simulink model "Beschl_self_geschaltet"  (R2021a)
settings: Solver=VariableStepAuto  StartTime=0.0  StopTime=20  RelTol=1e-3
values from neighbouring files (symbols this model uses):
  A = 1.7    [Parameter_Beschleunigen_Rueckschaltung.m]
  c_W = 0.32    [Parameter_Beschleunigen_Rueckschaltung.m]
  eta = 0.9    [Parameter_Beschleunigen_Rueckschaltung.m]
  F_R = 160    [Parameter_Beschleunigen_Rueckschaltung.m]
  i_A = 4.06    [Parameter_Beschleunigen_Rueckschaltung.m]
  i_G5 = 1.3    [Parameter_Beschleunigen_Rueckschaltung.m]
  m = 1600    [Parameter_Beschleunigen_Rueckschaltung.m]
  r_R = 0.291    [Parameter_Beschleunigen_Rueckschaltung.m]
  rho = 1.2    [Parameter_Beschleunigen_Rueckschaltung.m]
  v_0 = 60/3.6    (= 16.6666666667)    [Parameter_Beschleunigen_Rueckschaltung.m]
  v_max = r_R * omega_Rad_max    (= 37.5288777584)    [Parameter_Beschleunigen_Rueckschaltung.m]
  v_max_4 = r_R * omega_Rad_max_4    (= 23.2321624219)    [Parameter_Beschleunigen_Rueckschaltung.m]
libraries: simulink x2
settings Model: Creator=Kempk  LastModifiedBy=Kempk

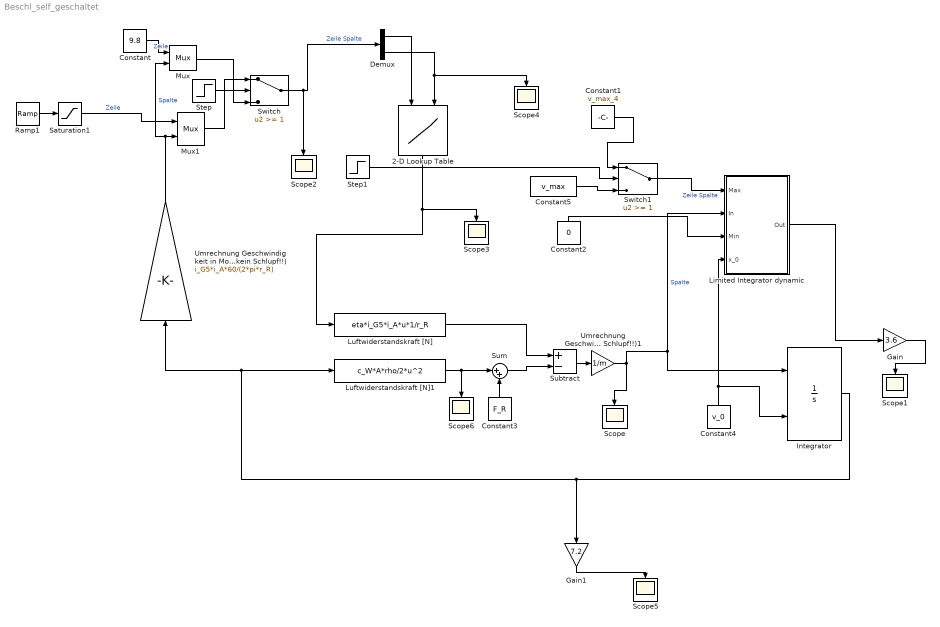
== system Beschl_self_geschaltet ==
  2-D Lookup Table : Lookup_n-D  BreakpointsForDimension1=KF_Motor(2:end,1)  BreakpointsForDimension2=KF_Motor(1,2:end)  Table=KF_Motor(2:end,2:end)  InternalRulePriority=Speed  RndMeth=Simplest  InputSameDT=on
      settings: InputPortMap=u0,u1
  Constant : Constant  Value=9.8
  Constant1 : Constant  Value=v_max_4
  Constant2 : Constant  Value=0
  Constant3 : Constant  Value=F_R
  Constant4 : Constant  Value=v_0
  Constant5 : Constant  Value=v_max
  Demux : Demux  Outputs=2
  Gain : Gain  Gain=3.6
  Gain1 : Gain  Gain=7.2
  Integrator : Integrator  InitialConditionSource=external  LimitOutput=on  UpperSaturationLimit=v_max
  Limited Integrator dynamic : Subsystem
  Luftwiderstandskraft [N] : Fcn  Expr=eta*i_G5*i_A*u*1/r_R
  Luftwiderstandskraft [N]1 : Fcn  Expr=c_W*A*rho/2*u^2
  Mux : Mux  Inputs=2
      settings: DisplayOption=signals
  Mux1 : Mux  Inputs=2
      settings: DisplayOption=signals
  Ramp1 : simulink/Sources/Ramp  slope=5000  start=3  InitialOutput=9.8
  Saturation1 : Saturate  UpperLimit=90  LowerLimit=9.8
  Scope{,1..6} (7 alike) : Scope
  Step : Step  Time=3  SampleTime=0
  Step1 : Step  Time=5  SampleTime=0
  Subtract : Sum  Inputs=+-
  Sum : Sum  Inputs=|++
  Switch : Switch  Threshold=1
  Switch1 : Switch  Threshold=1
  Umrechnung Geschwindigkeit in Motordrehzahl (kein Schlupf!!) : Gain  Gain=i_G5*i_A*60/(2*pi*r_R)
  Umrechnung Geschwindigkeit in Motordrehzahl (kein Schlupf!!)1 : Gain  Gain=1/m
  wires:
  Step/1 -> Switch/2
  Switch/1 -> Demux/1, Scope2/1  "Zeile Spalte"
  Luftwiderstandskraft [N]1/1 -> Sum/1, Scope6/1
  Constant3/1 -> Sum/2
  Sum/1 -> Subtract/2
  Luftwiderstandskraft [N]/1 -> Subtract/1
  2-D Lookup Table/1 -> Scope3/1, Luftwiderstandskraft [N]/1
  Integrator/1 -> Gain1/1, Umrechnung Geschwindigkeit in Motordrehzahl (kein Schlupf!!)/1, Luftwiderstandskraft [N]1/1
  Constant4/1 -> Limited Integrator dynamic/4(x_0), Integrator/2
  Constant/1 -> Mux/1  "Zeile"
  Saturation1/1 -> Mux1/1  "Zeile"
  Umrechnung Geschwindigkeit in Motordrehzahl (kein Schlupf!!)/1 -> Mux/2, Mux1/2  "Spalte"
  Demux/1 -> 2-D Lookup Table/1
  Demux/2 -> Scope4/1, 2-D Lookup Table/2
  Mux/1 -> Switch/3
  Mux1/1 -> Switch/1
  Gain/1 -> Scope1/1
  Ramp1/1 -> Saturation1/1
  Subtract/1 -> Umrechnung Geschwindigkeit in Motordrehzahl (kein Schlupf!!)1/1
  Umrechnung Geschwindigkeit in Motordrehzahl (kein Schlupf!!)1/1 -> Scope/1, Limited Integrator dynamic/2(In), Integrator/1  "Spalte"
  Limited Integrator dynamic/1(Out) -> Gain/1
  Constant2/1 -> Limited Integrator dynamic/3(Min)
  Step1/1 -> Switch1/2
  Switch1/1 -> Limited Integrator dynamic/1(Max)  "Zeile Spalte"
  Constant1/1 -> Switch1/1
  Constant5/1 -> Switch1/3
  Gain1/1 -> Scope5/1

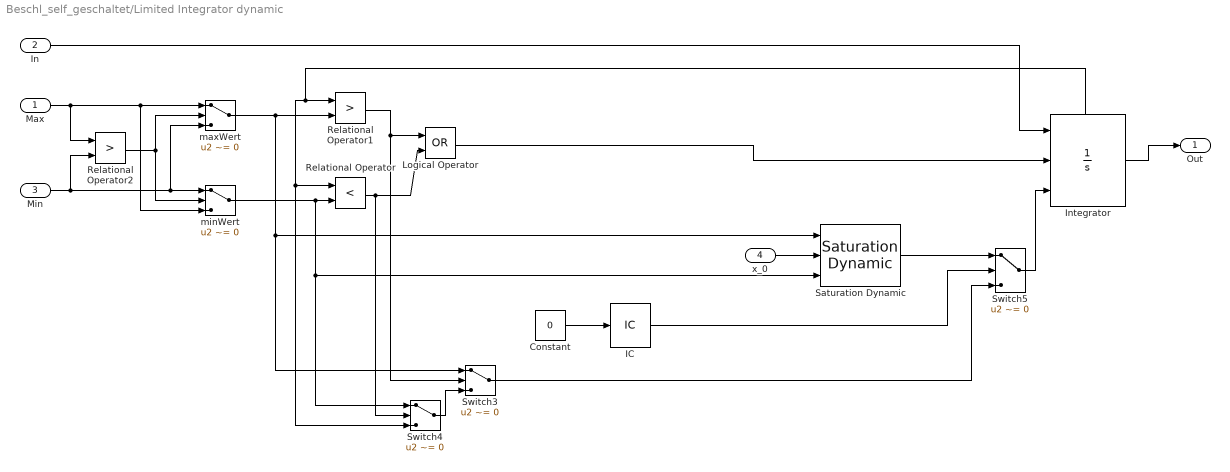
== system Beschl_self_geschaltet/Limited Integrator dynamic ==
  Max : Inport
  In : Inport  Port=2
  Min : Inport  Port=3
  x_0 : Inport  Port=4
  Constant : Constant  Value=0
  IC : InitialCondition
  Integrator : Integrator  ExternalReset=level  InitialConditionSource=external  ShowStatePort=on
  Logical Operator : Logic  Operator=OR  AllPortsSameDT=off  OutDataTypeStr=boolean
  Relational Operator : RelationalOperator  Operator=<  OutDataTypeStr=boolean  RndMeth=Nearest
  Relational Operator1 : RelationalOperator  Operator=>  OutDataTypeStr=boolean  RndMeth=Nearest
  Relational Operator2 : RelationalOperator  Operator=>  OutDataTypeStr=boolean  RndMeth=Nearest
  Saturation Dynamic : simulink/Discontinuities/Saturation Dynamic  OutMin=[]  OutMax=[]  OutDataTypeStr=Inherit: Same as second input  OutDataType=fixdt(1, 16)  OutScaling=2^-10  DoSatur=off
  Switch3 : Switch  Criteria=u2 ~= 0
  Switch4 : Switch  Criteria=u2 ~= 0
  Switch5 : Switch  Criteria=u2 ~= 0
  maxWert : Switch  Criteria=u2 ~= 0
  minWert : Switch  Criteria=u2 ~= 0
  Out : Outport
  wires:
  Integrator/1 -> Out/1
  maxWert/1 -> Relational Operator1/2, Switch3/1, Saturation Dynamic/1
  minWert/1 -> Relational Operator/2, Switch4/1, Saturation Dynamic/3
  Relational Operator1/1 -> Logical Operator/1, Switch3/2
  Relational Operator/1 -> Logical Operator/2, Switch4/2
  Max/1 -> minWert/3, maxWert/1, Relational Operator2/1
  Min/1 -> minWert/1, maxWert/3, Relational Operator2/2
  Relational Operator2/1 -> maxWert/2, minWert/2
  In/1 -> Integrator/1
  Integrator/State -> Relational Operator/1, Switch4/3, Relational Operator1/1
  Switch4/1 -> Switch3/3
  Logical Operator/1 -> Integrator/2
  Switch5/1 -> Integrator/3
  x_0/1 -> Saturation Dynamic/2
  Constant/1 -> IC/1
  Saturation Dynamic/1 -> Switch5/1
  IC/1 -> Switch5/2
  Switch3/1 -> Switch5/3
